simulink model "CodeEnLigne"  (Simulink 10.2)
settings: Solver=FixedStepDiscrete  StartTime=0.0  StopTime=10  RelTol=1e-3
model workspace (MAT data in the model file):
  M = Simulink.Parameter
  M.DataType = 'auto'
  M.Dimensions = [0 0]
libraries: commutil2 x4, commrandsrc3 x1, simulink_extras x1, dspsigops x1
settings Model: LogicAnalyzerSignalOrdering=6d594fe0-26bb-43f8-9994-1cd078bbf44d  Creator=iba  LastModifiedBy=mluser
settings SolverCC: AutoInsertRateTranBlk=on
settings DataIOCC: SaveFormat=Dataset  SignalLoggingSaveFormat=Dataset  SaveOutput=off  SignalLogging=off  SaveTime=off  ReturnWorkspaceOutputs=on
settings OptimizationCC: DefaultParameterBehavior=Inlined  LifeSpan=auto
settings DebuggingCC: AlgebraicLoopMsg=error  UnderspecifiedInitializationDetection=Simplified  MergeDetectMultiDrivingBlocksExec=error  SingleTaskRateTransMsg=warning  FcnCallInpInsideContextMsg=error  SFUnexpectedBacktrackingDiag=error  SFNoUnconditionalDefaultTransitionDiag=error  SFExecutionAtInitializationDiag=warning  ArithmeticOperatorsInVariantConditions=error
settings HardwareCC: ProdBitPerPointer=64  ProdBitPerSizeT=64  ProdBitPerPtrDiffT=64  ProdLargestAtomicFloat=Float  ProdIntDivRoundTo=Zero  ProdEndianess=LittleEndian  ProdWordSize=64  ProdHWDeviceType=Intel->x86-64 (Windows64)
settings ModelReferenceCC: PropagateSignalLabelsOutOfModel=on
settings SFSimCC: SimUseLocalCustomCode=on  CustomCodeUndefinedFunction=FilterOut
settings RTWCC: RTWUseLocalCustomCode=on
settings CodeAppCC: StateflowObjectComments=off
settings GRTTargetCC: TargetLangStandard=C99 (ISO)  CombineOutputUpdateFcns=on  GRTInterface=off
settings ConfigComp: CovMetricSettings=dwe  CovSaveCumulativeToWorkspaceVar=off  CovSaveSingleToWorkspaceVar=off  CovExternalEMLEnable=on

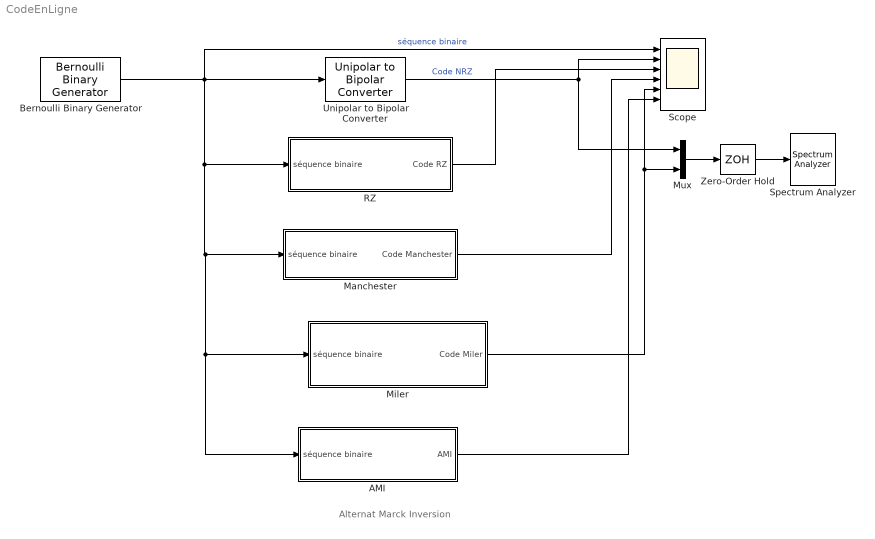
== system CodeEnLigne ==
  note: Alternat Marck Inversion
  AMI : Subsystem
  "Bernoulli Binary Generator " : commrandsrc3/Bernoulli Binary Generator  ProbabilityOfZero=0.5  SeedSource=Parameter  Seed=25  SampleTime=1  SamplesPerFrame=1  OutputDataType=double  SimulateUsing=Interpreted execution
  Manchester : Subsystem
  Miler : Subsystem
  Mux : Mux  Inputs=2
  RZ : Subsystem
  Scope : Scope  NumInputPorts=6
  Spectrum Analyzer : SpectrumAnalyzer
  Unipolar to Bipolar Converter : commutil2/Unipolar to Bipolar Converter  M=2  polarity=Positive  dataType=Inherit via internal rule
  Zero-Order Hold : ZeroOrderHold  SampleTime=0.1
  wires:
  "Bernoulli Binary Generator "/1 -> Unipolar to Bipolar Converter/1, Scope/1, AMI/1(séquence binaire), Miler/1(séquence binaire), Manchester/1(séquence binaire), RZ/1(séquence binaire)  "séquence binaire"
  Unipolar to Bipolar Converter/1 -> Mux/1, Scope/2  "Code NRZ"
  Zero-Order Hold/1 -> Spectrum Analyzer/1
  Mux/1 -> Zero-Order Hold/1
  RZ/1(Code RZ) -> Scope/3
  Manchester/1(Code Manchester) -> Scope/4
  Miler/1(Code Miler) -> Mux/2, Scope/5
  AMI/1(AMI) -> Scope/6

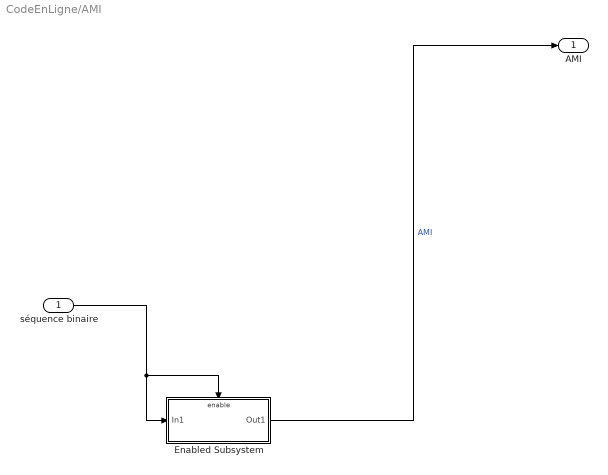
== system CodeEnLigne/AMI ==
  séquence binaire : Inport
  Enabled Subsystem : Subsystem  TreatAsAtomicUnit=on
  AMI : Outport
  wires:
  séquence binaire/1 -> Enabled Subsystem/1("In1 "), Enabled Subsystem/Enable
  Enabled Subsystem/1("Out1 ") -> AMI/1  "AMI"

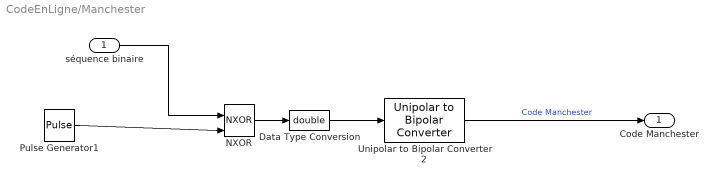
== system CodeEnLigne/Manchester ==
  séquence binaire : Inport
  "Data Type Conversion " : DataTypeConversion  OutDataTypeStr=double  LockScale=on
  NXOR : Logic  Operator=NXOR  IconShape=distinctive  AllPortsSameDT=off  OutDataTypeStr=boolean
  Pulse Generator1 : DiscretePulseGenerator
  Unipolar to Bipolar Converter 2 : commutil2/Unipolar to Bipolar Converter  M=2  polarity=Positive  dataType=Inherit via internal rule
  Code Manchester : Outport
  wires:
  Pulse Generator1/1 -> NXOR/2
  NXOR/1 -> "Data Type Conversion "/1
  séquence binaire/1 -> NXOR/1
  "Data Type Conversion "/1 -> Unipolar to Bipolar Converter 2/1
  Unipolar to Bipolar Converter 2/1 -> Code Manchester/1  "Code Manchester"

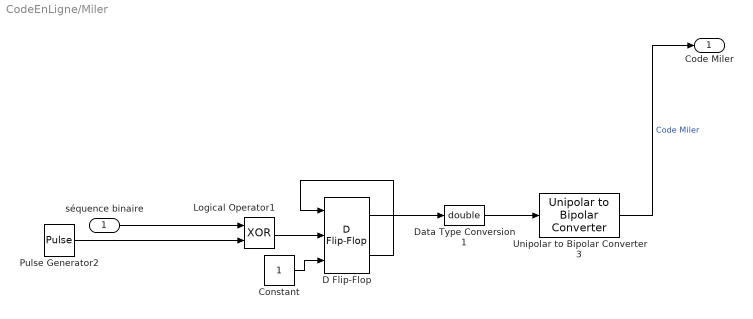
== system CodeEnLigne/Miler ==
  séquence binaire : Inport
  Constant : Constant
  D Flip-Flop : simulink_extras/Flip Flops/D Flip-Flop
  Data Type Conversion 1 : DataTypeConversion  OutDataTypeStr=double  LockScale=on
  Logical Operator1 : Logic  Operator=XOR  AllPortsSameDT=off  OutDataTypeStr=boolean
  Pulse Generator2 : DiscretePulseGenerator
  Unipolar to Bipolar Converter 3 : commutil2/Unipolar to Bipolar Converter  M=2  polarity=Positive  dataType=Inherit via internal rule
  Code Miler : Outport
  wires:
  séquence binaire/1 -> Logical Operator1/1
  Constant/1 -> D Flip-Flop/3
  Unipolar to Bipolar Converter 3/1 -> Code Miler/1  "Code Miler"
  Logical Operator1/1 -> D Flip-Flop/2
  Data Type Conversion 1/1 -> Unipolar to Bipolar Converter 3/1
  D Flip-Flop/2 -> D Flip-Flop/1
  Pulse Generator2/1 -> Logical Operator1/2
  D Flip-Flop/1 -> Data Type Conversion 1/1

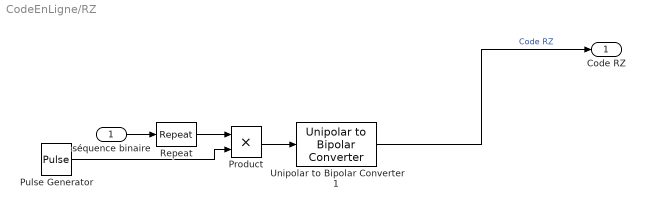
== system CodeEnLigne/RZ ==
  séquence binaire : Inport
  Product : Product
  Pulse Generator : DiscretePulseGenerator
  Repeat : dspsigops/Repeat  N=2  InputProcessing=Columns as channels (frame based)  RateOptions=Allow multirate processing  ic=0  mode=Unused parameter value
  Unipolar to Bipolar Converter 1 : commutil2/Unipolar to Bipolar Converter  M=2  polarity=Positive  dataType=Inherit via internal rule
  Code RZ : Outport
  wires:
  Unipolar to Bipolar Converter 1/1 -> Code RZ/1  "Code RZ"
  Pulse Generator/1 -> Product/2
  Repeat/1 -> Product/1
  Product/1 -> Unipolar to Bipolar Converter 1/1
  séquence binaire/1 -> Repeat/1

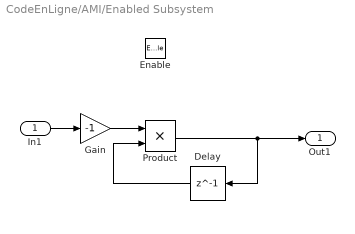
== system CodeEnLigne/AMI/Enabled Subsystem ==
  "In1 " : Inport
  Enable : EnablePort
  Delay : Delay  DelayLength=1  InitialCondition=-1
  Gain : Gain  Gain=-1
  Product : Product
  "Out1 " : Outport  OutputWhenDisabled=reset  InitialOutput=0
  wires:
  "In1 "/1 -> Gain/1
  Gain/1 -> Product/1
  Delay/1 -> Product/2
  Product/1 -> Delay/1, "Out1 "/1
